simulink model "sfcndemo_cppcount"  (R2020b)
settings: Solver=FixedStepDiscrete  StartTime=0.0  StopTime=10  FixedStep=1  RelTol=1e-3  EnableMultiTasking=on
Description:
  | Bringing in C++ Code into a C++ S-function Including Code Generation Support
settings Model: ExtModeTrigMode=oneshot  ExtModeArmWhenConnect=off  ExtModeAutoUpdateStatusClock=off  Creator=The MathWorks, Inc.  LastModifiedBy=yinti
settings DataIOCC: SaveFormat=Array  SaveOutput=off  SignalLogging=off  SaveTime=off  SignalLoggingName=logsOut
settings OptimizationCC: ExpressionDepthLimit=2147483647  StateBitsets=on  DataBitsets=on  InitFltsAndDblsToZero=on  LifeSpan=inf  BufferReusableBoundary=off
settings DebuggingCC: SaveWithParameterizedLinksMsg=none  SignalResolutionControl=TryResolveAllWithWarning  MultiTaskDSMMsg=warning  MultiTaskCondExecSysMsg=none  SigSpecEnsureSampleTimeMsg=none  FcnCallInpInsideContextMsg=warning  AllowSymbolicDim=off  StateNameClashWarn=warning  SFUnexpectedBacktrackingDiag=warning  SFNoUnconditionalDefaultTransitionDiag=warning  SFExecutionAtInitializationDiag=none  ArithmeticOperatorsInVariantConditions=warning
settings HardwareCC: ProdBitPerPointer=32  ProdBitPerSizeT=32  ProdBitPerPtrDiffT=32  ProdLargestAtomicFloat=None  ProdIntDivRoundTo=Undefined  ProdEndianess=Unspecified  ProdWordSize=32  ProdHWDeviceType=Specified  TargetHWDeviceType=32-bit Generic  ProdEqTarget=off
settings ModelReferenceCC: PropagateSignalLabelsOutOfModel=off
settings SFSimCC: SimUseLocalCustomCode=off  CustomCodeUndefinedFunction=UseInterfaceOnly  SimTargetLang=C++
settings RTWCC: GenerateReport=on  RTWVerbose=off  RTWUseLocalCustomCode=off  CustomSourceCode="#include \"sfun_cppcount_cpp.h\""  CustomInclude="\"$matlabroot$/toolbox/simulink/simdemos/simfeatures/include\""  LaunchReport=on  TargetLang=C++
settings CodeAppCC: ForceParamTrailComments=on  StateflowObjectComments=on
settings GRTTargetCC: TargetFcnLib=ansi_tfl_tmw.mat  TargetLangStandard=C89/C90 (ANSI)  CombineOutputUpdateFcns=off  GRTInterface=on
settings ConfigComp: CovMetricSettings=dw  CovSaveCumulativeToWorkspaceVar=on  CovSaveSingleToWorkspaceVar=on  CovExternalEMLEnable=off

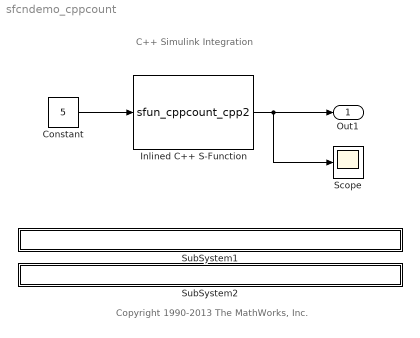
== system sfcndemo_cppcount ==
  note: C++ Simulink Integration
  note: Copyright 1990-2013 The MathWorks, Inc.
  Constant : Constant  Value=5
  Inlined C++ S-Function : S-Function  FunctionName=sfun_cppcount_cpp2  SFunctionDeploymentMode=off  EnableBusSupport=off
      mask Display: disp('Inlined C++\nS-Function');
  Scope : Scope
  SubSystem1 : Subsystem  mask{filename=sfun_cppcount_cpp.cpp}
      mask init:
      | x=sfundemo_maskdisp;
      settings: AttributesFormatString=\n  OpenFcn=sfundemo_openfcn
      mask Display: disp(x);
  SubSystem2 : Subsystem  mask{filename=sfun_cppcount_cpp.h}
      mask init:
      | x=sfundemo_maskdisp;
      settings: AttributesFormatString=\n  OpenFcn=sfundemo_openfcn
      mask Display: disp(x);
  Out1 : Outport  VectorParamsAs1DForOutWhenUnconnected=off
  wires:
  Inlined C++ S-Function/1 -> Out1/1, Scope/1
  Constant/1 -> Inlined C++ S-Function/1

== system sfcndemo_cppcount/SubSystem1 ==

== system sfcndemo_cppcount/SubSystem2 ==
